simulink model "model"  (R2015a)
settings: Solver=ode45  StartTime=0.0  StopTime=500  RelTol=1e-3
values from neighbouring files (symbols this model uses):
  DR = val(:,2)    [runfirst.m]
  HEIGHT = val(:,3)    [runfirst.m]
  PITCH = val(:,4)    [runfirst.m]
  TIME = val(:,1)    [runfirst.m]    (also in shuttle_model.m = y(:,1))
undefined symbols (not defined in the file or in its folder): Earth, WGS84
libraries: simulink x2, aerolibtransform2 x1, aerolibfltsims x1
settings Model: Creator=vinay  LastModifiedBy=vinay

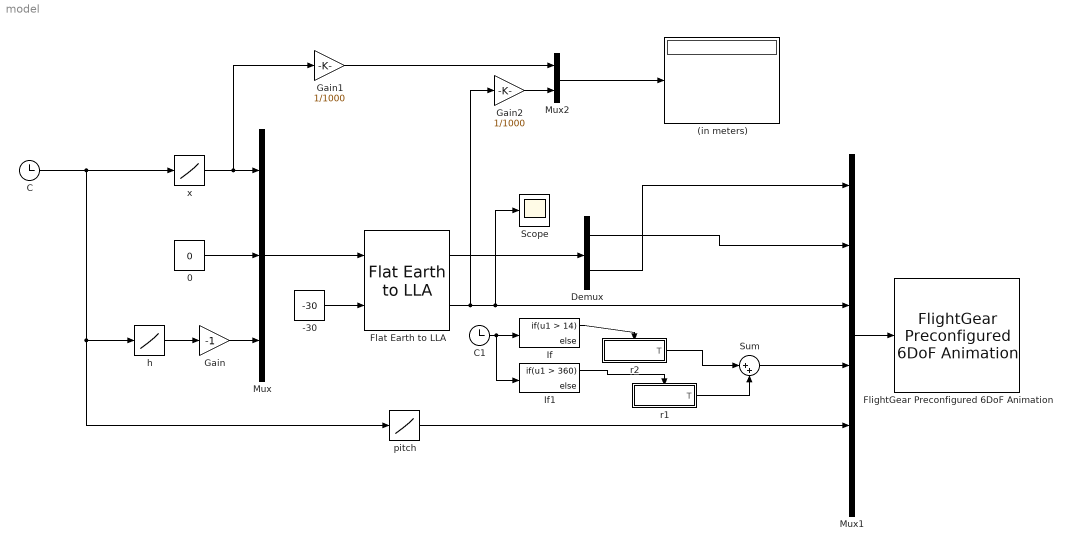
== system model ==
  (in meters) : Display
  -30 : Constant  Value=-30
  0 : Constant  Value=0
  C : Clock
  C1 : Clock
  Demux : Demux  Outputs=2
  Flat Earth to LLA : aerolibtransform2/Flat Earth to LLA  units=Metric (MKS)  ptype=Earth (WGS84)  F=1/298.257223563  R=6378137  LL0=[28.608397 -80.604345]  psi=0
  FlightGear Preconfigured 6DoF Animation : aerolibfltsims/FlightGear Preconfigured 6DoF Animation  xFlightGearVersion=v3.0  DestinationIpAddress=127.0.0.1  DestinationPort=5502  SampleTime=1/150
  Gain : Gain  Gain=-1
  Gain1 : Gain  Gain=1/1000
  Gain2 : Gain  Gain=1/1000
  If : If  IfExpression=u1 > 14
  If1 : If  IfExpression=u1 > 360
  Mux : Mux  Inputs=3
  Mux1 : Mux  Inputs=6
  Mux2 : Mux  Inputs=2
  Scope : Scope
      settings: YMin=0  YMax=90000
  Sum : Sum  Inputs=|++
  h : Lookup  InputValues=TIME  Table=HEIGHT  LookUpMeth=Interpolation-Use End Values  SaturateOnIntegerOverflow=on
  pitch : Lookup  InputValues=TIME  Table=PITCH  LookUpMeth=Interpolation-Use End Values  SaturateOnIntegerOverflow=on
  r1 : Subsystem  TreatAsAtomicUnit=on
  r2 : Subsystem  TreatAsAtomicUnit=on
  x : Lookup  InputValues=TIME  Table=DR  LookUpMeth=Interpolation-Use End Values  SaturateOnIntegerOverflow=on
  wires:
  Flat Earth to LLA/1 -> Demux/1
  x/1 -> Gain1/1, Mux/1
  Mux/1 -> Flat Earth to LLA/1
  0/1 -> Mux/2
  h/1 -> Gain/1
  Flat Earth to LLA/2 -> Gain2/1, Scope/1, Mux1/3
  pitch/1 -> Mux1/5
  Mux1/1 -> FlightGear Preconfigured 6DoF Animation/1
  Gain/1 -> Mux/3
  -30/1 -> Flat Earth to LLA/2
  Demux/1 -> Mux1/2
  Demux/2 -> Mux1/1
  C/1 -> pitch/1, h/1, x/1
  If/1 -> r2/Action
  C1/1 -> If1/1, If/1
  Sum/1 -> Mux1/4
  If1/1 -> r1/Action
  r2/1(T) -> Sum/1
  r1/1(T) -> Sum/2
  Mux2/1 -> (in meters)/1
  Gain1/1 -> Mux2/1
  Gain2/1 -> Mux2/2

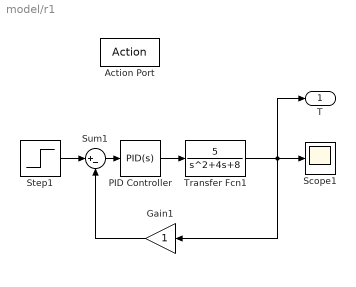
== system model/r1 ==
  Action Port : ActionPort  ActionType=then
  Gain1 : Gain
  PID Controller : simulink/Continuous/PID Controller  Controller=PID  TimeDomain=Continuous-time  SampleTime=-1  IntegratorMethod=Forward Euler  FilterMethod=Forward Euler  Form=Parallel  UseFilter=on  ControllerParametersSource=internal  P=1  I=1  D=0.2  N=100  InitialConditionSource=internal  InitialConditionForIntegrator=0  InitialConditionForFilter=0  ExternalReset=none  LimitOutput=off  UpperSaturationLimit=inf  LowerSaturationLimit=-inf  LinearizeAsGain=on  AntiWindupMode=none  Kb=1  TrackingMode=off  Kt=1  PParamMin=[]  PParamMax=[]  IParamMin=[]  IParamMax=[]  DParamMin=[]  DParamMax=[]  NParamMin=[]  NParamMax=[]  KbParamMin=[]  KbParamMax=[]  KtParamMin=[]  KtParamMax=[]  POutMin=[]  POutMax=[]  IOutMin=[]  IOutMax=[]  DOutMin=[]  DOutMax=[]  NOutMin=[]  NOutMax=[]  KbOutMin=[]  KbOutMax=[]  KtOutMin=[]  KtOutMax=[]  IntegratorOutMin=[]  IntegratorOutMax=[]  FilterOutMin=[]  FilterOutMax=[]  SumOutMin=[]  SumOutMax=[]  SumI1OutMin=[]  SumI1OutMax=[]  SumI2OutMin=[]  SumI2OutMax=[]  SumI3OutMin=[]  SumI3OutMax=[]  SumDOutMin=[]  SumDOutMax=[]  SaturationOutMin=[]  SaturationOutMax=[]  IntegratorContinuousStateAttributes=''  IntegratorStateMustResolveToSignalObject=off  IntegratorRTWStateStorageClass=Auto  FilterContinuousStateAttributes=''  FilterStateMustResolveToSignalObject=off  FilterRTWStateStorageClass=Auto  DifferentiatorICPrevScaledInput=0  DifferentiatorOutMin=[]  DifferentiatorOutMax=[]
  Scope1 : Scope
      settings: YMin=0.25  YMax=1.75
  Step1 : Step  Time=0  After=3.14159  SampleTime=0  ZeroCross=off
  Sum1 : Sum  Inputs=|+-
  Transfer Fcn1 : TransferFcn  Numerator=[5]  Denominator=[1 4 8]
  T : Outport
  wires:
  Transfer Fcn1/1 -> Gain1/1, T/1, Scope1/1
  Sum1/1 -> PID Controller/1
  Step1/1 -> Sum1/1
  Gain1/1 -> Sum1/2
  PID Controller/1 -> Transfer Fcn1/1

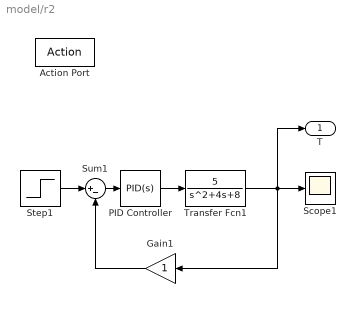
== system model/r2 ==
  Action Port : ActionPort  ActionType=then
  Gain1 : Gain
  PID Controller : simulink/Continuous/PID Controller  Controller=PID  TimeDomain=Continuous-time  SampleTime=-1  IntegratorMethod=Forward Euler  FilterMethod=Forward Euler  Form=Parallel  UseFilter=on  ControllerParametersSource=internal  P=1  I=1  D=0.2  N=100  InitialConditionSource=internal  InitialConditionForIntegrator=0  InitialConditionForFilter=0  ExternalReset=none  LimitOutput=off  UpperSaturationLimit=inf  LowerSaturationLimit=-inf  LinearizeAsGain=on  AntiWindupMode=none  Kb=1  TrackingMode=off  Kt=1  PParamMin=[]  PParamMax=[]  IParamMin=[]  IParamMax=[]  DParamMin=[]  DParamMax=[]  NParamMin=[]  NParamMax=[]  KbParamMin=[]  KbParamMax=[]  KtParamMin=[]  KtParamMax=[]  POutMin=[]  POutMax=[]  IOutMin=[]  IOutMax=[]  DOutMin=[]  DOutMax=[]  NOutMin=[]  NOutMax=[]  KbOutMin=[]  KbOutMax=[]  KtOutMin=[]  KtOutMax=[]  IntegratorOutMin=[]  IntegratorOutMax=[]  FilterOutMin=[]  FilterOutMax=[]  SumOutMin=[]  SumOutMax=[]  SumI1OutMin=[]  SumI1OutMax=[]  SumI2OutMin=[]  SumI2OutMax=[]  SumI3OutMin=[]  SumI3OutMax=[]  SumDOutMin=[]  SumDOutMax=[]  SaturationOutMin=[]  SaturationOutMax=[]  IntegratorContinuousStateAttributes=''  IntegratorStateMustResolveToSignalObject=off  IntegratorRTWStateStorageClass=Auto  FilterContinuousStateAttributes=''  FilterStateMustResolveToSignalObject=off  FilterRTWStateStorageClass=Auto  DifferentiatorICPrevScaledInput=0  DifferentiatorOutMin=[]  DifferentiatorOutMax=[]
  Scope1 : Scope
      settings: TimeRange=11  YMin=0  YMax=3.5  SaveName=ScopeData2
  Step1 : Step  Time=0  After=3.14159  SampleTime=0  ZeroCross=off
  Sum1 : Sum  Inputs=|+-
  Transfer Fcn1 : TransferFcn  Numerator=[5]  Denominator=[1 4 8]
  T : Outport
  wires:
  Transfer Fcn1/1 -> Gain1/1, T/1, Scope1/1
  Sum1/1 -> PID Controller/1
  Step1/1 -> Sum1/1
  Gain1/1 -> Sum1/2
  PID Controller/1 -> Transfer Fcn1/1
